simulink library "SafetyModule"  (R2016b)
settings: Solver=VariableStepAuto  StartTime=0.0  StopTime=10.0  RelTol=1e-3
undefined symbols (not defined in the file or in its folder): ExoskeletonState
libraries: ErrorDetector x1, ErrorReactionHandler x1
settings Model: Creator=march  LastModifiedBy=march

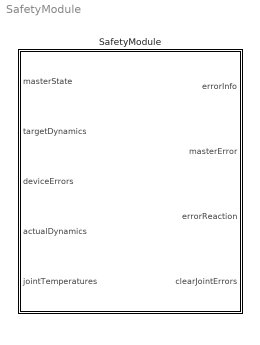
== system SafetyModule ==
  SafetyModule : Subsystem

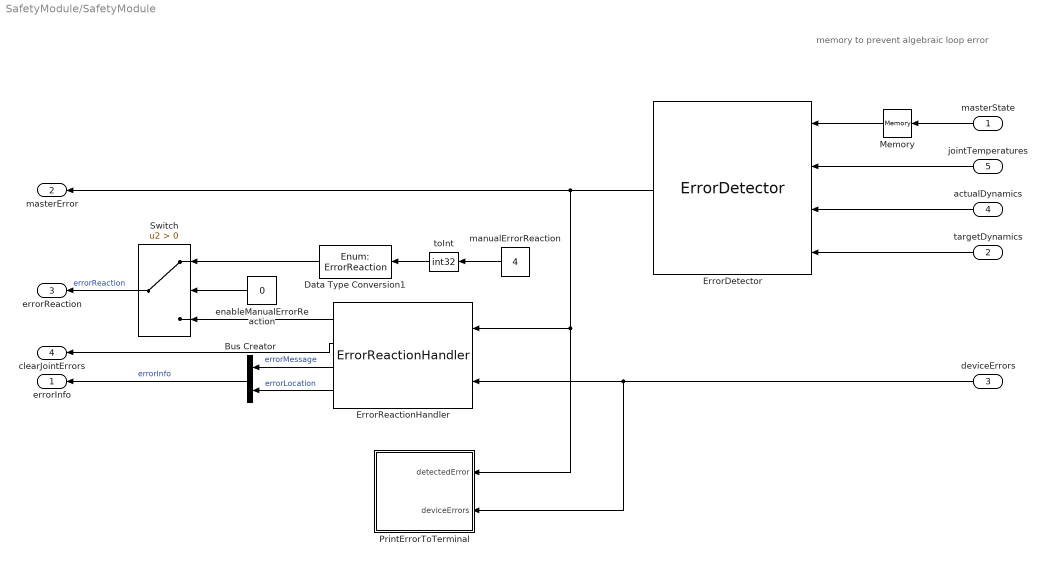
== system SafetyModule/SafetyModule ==
  note: memory to prevent algebraic loop error
  masterState : Inport
  targetDynamics : Inport  Port=2
  deviceErrors : Inport  Port=3
  actualDynamics : Inport  Port=4
  jointTemperatures : Inport  Port=5
  Bus Creator : BusCreator  Inputs=2  OutDataTypeStr=Bus: ErrorInfo
  Data Type Conversion1 : DataTypeConversion  OutDataTypeStr=Enum: ErrorReaction
  ErrorDetector : ErrorDetector/ErrorDetector
  ErrorReactionHandler : ErrorReactionHandler/ErrorReactionHandler
  Memory : Memory  X0=ExoskeletonState.FULLMANUAL
  PrintErrorToTerminal : Subsystem
  Switch : Switch  Criteria=u2 > Threshold
  enableManualErrorReaction : Constant  Value=0
  manualErrorReaction : Constant  Value=4
  toInt : DataTypeConversion  OutDataTypeStr=int32
  errorInfo : Outport  OutDataTypeStr=Bus: ErrorInfo
  masterError : Outport  Port=2
  errorReaction : Outport  Port=3
  clearJointErrors : Outport  Port=4
  wires:
  Bus Creator/1 -> errorInfo/1  "errorInfo"
  ErrorReactionHandler/4 -> Bus Creator/2  "errorLocation"
  ErrorReactionHandler/3 -> Bus Creator/1  "errorMessage"
  deviceErrors/1 -> PrintErrorToTerminal/2(deviceErrors), ErrorReactionHandler/2
  actualDynamics/1 -> ErrorDetector/3
  masterState/1 -> Memory/1
  jointTemperatures/1 -> ErrorDetector/2
  ErrorDetector/1 -> masterError/1, PrintErrorToTerminal/1(detectedError), ErrorReactionHandler/1
  ErrorReactionHandler/2 -> clearJointErrors/1
  targetDynamics/1 -> ErrorDetector/4
  ErrorReactionHandler/1 -> Switch/3
  Switch/1 -> errorReaction/1  "errorReaction"
  manualErrorReaction/1 -> toInt/1
  toInt/1 -> Data Type Conversion1/1
  Data Type Conversion1/1 -> Switch/1
  enableManualErrorReaction/1 -> Switch/2
  Memory/1 -> ErrorDetector/1

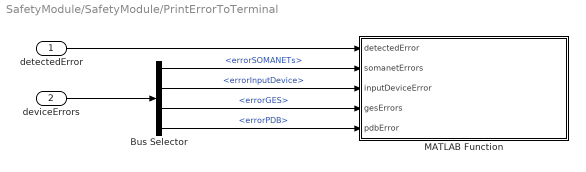
== system SafetyModule/SafetyModule/PrintErrorToTerminal ==
  detectedError : Inport
  deviceErrors : Inport  Port=2
  Bus Selector : BusSelector  OutputSignals=errorSOMANETs,errorInputDevice,errorGES,errorPDB
  MATLAB Function : MATLAB Function  TreatAsAtomicUnit=on
  wires:
  Bus Selector/1 -> MATLAB Function/2(somanetErrors)  "<errorSOMANETs>"
  Bus Selector/2 -> MATLAB Function/3(inputDeviceError)  "<errorInputDevice>"
  Bus Selector/3 -> MATLAB Function/4(gesErrors)  "<errorGES>"
  Bus Selector/4 -> MATLAB Function/5(pdbError)  "<errorPDB>"
  deviceErrors/1 -> Bus Selector/1
  detectedError/1 -> MATLAB Function/1(detectedError)

== matlab function SafetyModule/PrintErrorToTerminal/MATLAB Function ==
  data: detectedError input; somanetErrors input; inputDeviceError input; gesErrors input; pdbError input
function printErrorToTerminal(detectedError, somanetErrors, inputDeviceError, gesErrors, pdbError)
% wrapper for printErrorToTerminal
printErrorToTerminal(detectedError, somanetErrors, inputDeviceError, gesErrors, pdbError);
end
